simulink model "shiyankongzhixitong"  (R2023b)
settings: Solver=VariableStepAuto  StartTime=0.0  StopTime=2  RelTol=1e-3
libraries: spspowerguiLib x1
settings Model: Creator=ASUS  LastModifiedBy=ASUS

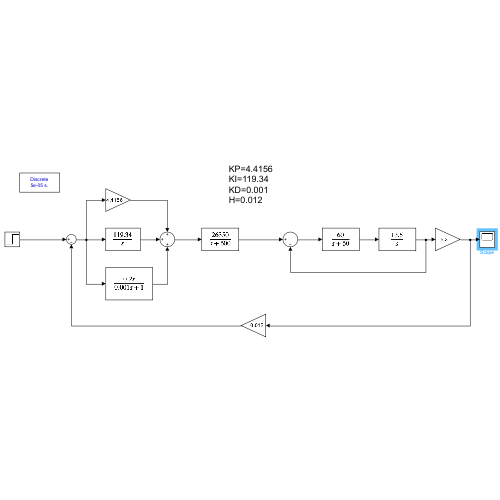
[thumbnail: Simulink's stored preview of the top-level diagram]
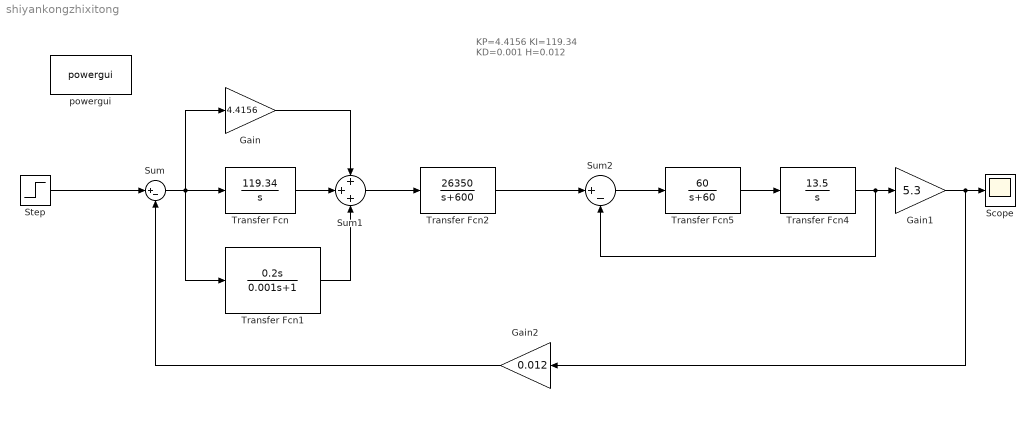
== system shiyankongzhixitong ==
  note: KP=4.4156
      | KI=119.34
      | KD=0.001
      | H=0.012
  Gain : Gain  Gain=4.4156
  Gain1 : Gain  Gain=5.3
  Gain2 : Gain  Gain=0.012
  Scope : Scope
  Step : Step  SampleTime=0
  Sum : Sum  Inputs=|+-
  Sum1 : Sum  Inputs=+++
  Sum2 : Sum  Inputs=|+-
  Transfer Fcn : TransferFcn  Numerator=[119.34]  Denominator=[1 0]
  Transfer Fcn1 : TransferFcn  Numerator=[0.2 0]  Denominator=[0.001 1]
  Transfer Fcn2 : TransferFcn  Numerator=[26350]  Denominator=[1 600]
  Transfer Fcn4 : TransferFcn  Numerator=[13.5]  Denominator=[1 0]
  Transfer Fcn5 : TransferFcn  Numerator=[60]  Denominator=[1 60]
  powergui : spspowerguiLib/powergui  Priority=1  SimulationMode=Discrete  SampleTime=50e-6  frequency=60  Iterations=50  frequencyindice=60  Pbase=100e6  ErrMax=1e-4  UnitsV=kV  UnitsW=MW  buscounter=0  FunctionMessages=off  echomessages=off  EnableUseOfTLC=off  CurrentSourceSwitches=off  DisableSnubberDevices=off  DisableRonSwitches=off  DisableVfSwitches=off  DisplayEquations=off  AutomaticDiscreteSolvers=off  SolverType=Tustin/Backward Euler (TBE)  Interpol=off  ExternalGateDelay=off  methode=off  Ts=100  x0status=blocks  SPID=on  SwTol=0  HookPort=off  NonlinearTolerance=1e-4  nMaxIteration=100  ContinueOnMaxIteration=off  RestoreLinks=warning  ResistiveCurrentMeasurement=off  Frange=[0:2:500]  Ylog=off  Xlog=on  ShowGrid=off  save=off  variable=ZData  structure=0  ZoomFFT=off  StartTime=0.0  cycles=1  DisplayStyle=1  fundamental=60  FreqAxis=off  MaxFrequency=1000  frequencyindicesteady=1  RmsSteady=1  display=off
  wires:
  Step/1 -> Sum/1
  Sum/1 -> Transfer Fcn1/1, Transfer Fcn/1, Gain/1
  Transfer Fcn/1 -> Sum1/2
  Gain/1 -> Sum1/1
  Transfer Fcn1/1 -> Sum1/3
  Sum1/1 -> Transfer Fcn2/1
  Gain1/1 -> Gain2/1, Scope/1
  Transfer Fcn4/1 -> Sum2/2, Gain1/1
  Transfer Fcn5/1 -> Transfer Fcn4/1
  Sum2/1 -> Transfer Fcn5/1
  Transfer Fcn2/1 -> Sum2/1
  Gain2/1 -> Sum/2
